simulink model "RoboticFish_Maneuverability_model"  (R2022b)
settings: Solver=ode4  StartTime=0.0  StopTime=50  FixedStep=0.01  RelTol=1e-3  EnableMultiTasking=on
libraries: sharedutil x15, matrix_library x1, dspvision x1, vrlib x1
(part 1 of 3)
settings Model: Creator=Waqas Ali Waqar  LastModifiedBy=Administrator
settings SolverCC: ConcurrentTasks=on  AlgebraicLoopSolver=TrustRegion  AutoInsertRateTranBlk=on  InsertRTBMode=Never (minimum delay)
settings DataIOCC: SaveFormat=StructureWithTime
settings OptimizationCC: BlockReduction=off  OptimizeBlockIOStorage=off  BufferReuse=off  GlobalBufferReuse=off  ExpressionFolding=off  PassReuseOutputArgsThreshold=0  LocalBlockOutputs=off  OptimizeBlockOrder=speed  OptimizeDataStoreBuffers=off  BusAssignmentInplaceUpdate=off
settings DebuggingCC: ParameterTunabilityLossMsg=error  UnconnectedInputMsg=warning  UnconnectedOutputMsg=warning  UnconnectedLineMsg=warning
settings HardwareCC: ProdBitPerPointer=32  ProdBitPerSizeT=32  ProdBitPerPtrDiffT=32  ProdLargestAtomicFloat=None  ProdWordSize=32  ProdLongLongMode=on  ProdHWDeviceType=Generic->32-bit x86 compatible
settings ModelReferenceCC: EnableRefExpFcnMdlSchedulingChecks=on
settings SFSimCC: MATLABDynamicMemAlloc=off  CustomCodeUndefinedFunction=UseInterfaceOnly
settings RTWCC: GenerateReport=on  RTWVerbose=off  LaunchReport=on  RTWCompilerOptimization=on  DLArmComputeVersion=19.05
settings CodeAppCC: ForceParamTrailComments=on  OperatorAnnotations=on
settings GRTTargetCC: TargetLangStandard=C89/C90 (ANSI)

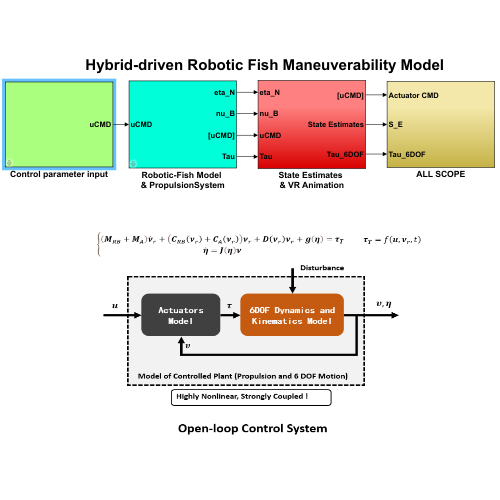
[thumbnail: Simulink's stored preview of the top-level diagram]
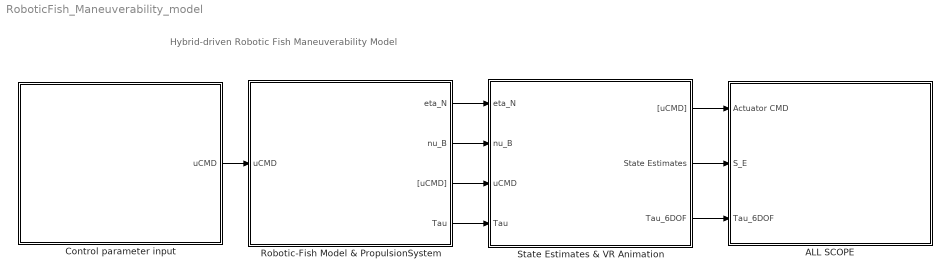
== system RoboticFish_Maneuverability_model ==
  note: Hybrid-driven Robotic Fish Maneuverability Model
  ALL SCOPE : Subsystem
  Control parameter input : Subsystem  mask{PropChoice=on, uHT1=500, uHT2=0, uVT1=1000, FinChoice=off, f_HT3=2, Thetastr_HT3=0, uVT2=60, uVT3=60}
      mask prompts: PropChoice "Choice Propeller Actuators"; uHT1 "uHT1(rpm)"; uHT2 "uHT2(rpm)"; uVT1 "uVT1(rpm)"; FinChoice "Choice Fin Actuators"; f_HT3 "f_HT3(Hz)"; Thetastr_HT3 "Thetastr_HT3(deg)"; uVT2 "uVT2(deg)"; uVT3 "uVT3(deg)"
      mask Callback PropChoice:
      | usePropChoice = get_param(gcbh,'PropChoice');
      | mask_v = get_param(gcbh,'MaskVisibilities');
      | if strcmp('on',usePropChoice)
      |    mask_v{2}='on';
      |    mask_v{3}='on';
      |    mask_v{4}='on';
      | else
      |    mask_v{2}='off';
      |    mask_v{3}='off';
      |    mask_v{4}='off';
      | end
      | set_param(gcbh,'MaskVisibilities',mask_v);
      mask Callback FinChoice:
      | useFinChoice = get_param(gcbh,'FinChoice');
      | mask_v = get_param(gcbh,'MaskVisibilities');
      | if strcmp('on',useFinChoice)
      |    mask_v{6}='on';
      |    mask_v{7}='on';
      |    mask_v{8}='on';
      |    mask_v{9}='on';
      | else
      |    mask_v{6}='off';
      |    mask_v{7}='off';
      |    mask_v{8}='off';
      |    mask_v{9}='off';
      | end
      | set_param(gcbh,'MaskVisibilities',mask_v);
  Robotic-Fish Model & PropulsionSystem : Subsystem  mask{Ig=[0.5025 0 0;0 4.8344 0;0 0 4.9297], m=48, rho=1000, W=470.4, B=470.4, rG_B=[0;0;0], rB_B=[0;0;-0.2], DL=diag([-1.1;2.559;-1.458;0.000811;-0.382;-1.621]), S=0.103, Amp=0.182, ld=0.239, kw=1, a2=1.905, a1=-0.7047, a0=0.01797, b2=2.081, b1=-0.3937, b0=0.09809, c2=20.652, d2=17.102, phisurge=1.0158, phisway=3.792, phiyaw=13.362, cL=0.5, xfin=0.192, yfin=0.225, zfin=0.083, alpha=0, Sfin=0.0121, e1=[1;0;0], r1=[-0.107;-0.222;0], e2=[1;0;0], r2=[-0.107;0.222;0], e3=[0;0;1], r3=[-0.143;0;-0.021], D=0.0762}
      mask prompts: Ig "Inertia Tensor Ig:"; m "Mass m:"; rho "Seawater Density rho:"; W "Weight"; B "Buoyancy"; DL "Linear Damping Matrix"; S "Tail area S (m^2)"; Amp "Tail-beat amplitude Amp (m)"; ld "Distance from the center of hydrodynamic action of the tail to the origin ld (m)"; kw "Adjustment coefficient kw"; cL "fin lift coefficient  cL:"; xfin "fin axial position xfin:"; yfin "fin axial position yfin:"; zfin "fin axial position zfin:"; alpha "fin flutter angle alpha"; Sfin "fin platform area Sfin:"; e1 "e1 (HT1):"; r1 "r1 (HT1):"; e2 "e2 (HT2 ):"; r2 "r2 (HT2):"; e3 "e3 (VT1):"; r3 "r3 (VT1):"; D "Diameter"
      mask init:
      | %%%%%%%%%%%%%%%%%%%%%%%%%%%%%%%%%%%%%%%%%%%%%%%%%%%%%%%
      | %%%%%%%%%%%%%%%%%%%  动力学  %%%%%%%%%%%%%%%%%%%%%%%%
      | %%%%%%%%%%%%%%%%%%%%%%%%%%%%%%%%%%%%%%%%%%%%%%%%%%%%%%%
      | 
      | % 惯性张量与广义质量矩阵
      | Ib = Ig-m*skewsymm(rG_B)*skewsymm(rG_B);
      | MRB = [m*eye(3,3) -m*skewsymm(rG_B); m*skewsymm(rG_B) Ib];
      | 
      | % 附加质量系数
      | X_udot = -7.445;
      | Y_vdot = -63.087;
      | Z_wdot = -63.087;
      | K_pdot = 0;
      | M_qdot = -4.824;
      | N_rdot = -4.824;
      | 
      | 
      | % 附加质量矩阵
      | MA = -diag([X_udot;Y_vdot;Z_wdot;K_pdot;M_qdot;N_rdot]);
      | 
      | % 总的广义质量矩阵（包括附加质量矩阵）
      | M = MRB + MA;
      | inv_M = inv(M);
      | M11 = MA(1:3,1:3);    M12 = MA(1:3,4:6);
      | M21 = MA(4:6,1:3);    M22 = MA(4:6,4:6);
      | 
      | %% 粘性水动力系数
      | X_uu = -3.886;
      | Y_vv = -113;
      | Z_ww = -71.631;
      | K_pp = -0.158;
      | M_qq = -2.127;
      | N_rr = -22.381;
      | 
      | dQ = ([X_uu;Y_vv;Z_ww;K_pp;M_qq;N_rr]);
      | 
      | 
      | %%%%%%%%%%%%%%%%%%%%%%%%%%%%%%%%%%%%%%%%%%%%%%%%%%%%%%%
      | %%%%%%%%%%%%%%%%%%%  PROP HT1 HT2 VT1  %%%%%%%%%%%%%%%%
      | %%%%%%%%%%%%%%%%%%%%%%%%%%%%%%%%%%%%%%%%%%%%%%%%%%%%%%%
      | 
      | K1 = rho*D*D*D;
      | K2 = rho*D*D*D;
      | K3 = rho*D*D*D;
      | HT_prop = [e1 e2;skewsymm(r1)*e1 skewsymm(r2)*e2]*diag([K1;K2]);
      | VT_prop = [e3 ;skewsymm(r3)*e3 ]*K3;
      mask DialogControl DescGroupVar Prompt: Robotic Fish Paramteres
      mask DialogControl Container14 Prompt: Robotic Fish Parameters
      mask DialogControl Container17 Prompt: Caudal Fin Parameters
      mask DialogControl Container18 Prompt: Pectoral Fins Parameters
      mask DialogControl Container19 Prompt: Thrusters Parameters
  State Estimates & VR Animation : Subsystem
  wires:
  Robotic-Fish Model & PropulsionSystem/2(nu_B) -> State Estimates & VR Animation/2(nu_B)
  Robotic-Fish Model & PropulsionSystem/1(eta_N) -> State Estimates & VR Animation/1(eta_N)
  Control parameter input/1(uCMD) -> Robotic-Fish Model & PropulsionSystem/1(uCMD)
  Robotic-Fish Model & PropulsionSystem/3("[uCMD]") -> State Estimates & VR Animation/3(uCMD)
  State Estimates & VR Animation/2(State Estimates) -> ALL SCOPE/2(S_E)
  State Estimates & VR Animation/1("[uCMD]") -> ALL SCOPE/1(Actuator CMD)
  Robotic-Fish Model & PropulsionSystem/4(Tau) -> State Estimates & VR Animation/4(Tau)
  State Estimates & VR Animation/3(Tau_6DOF) -> ALL SCOPE/3(Tau_6DOF)

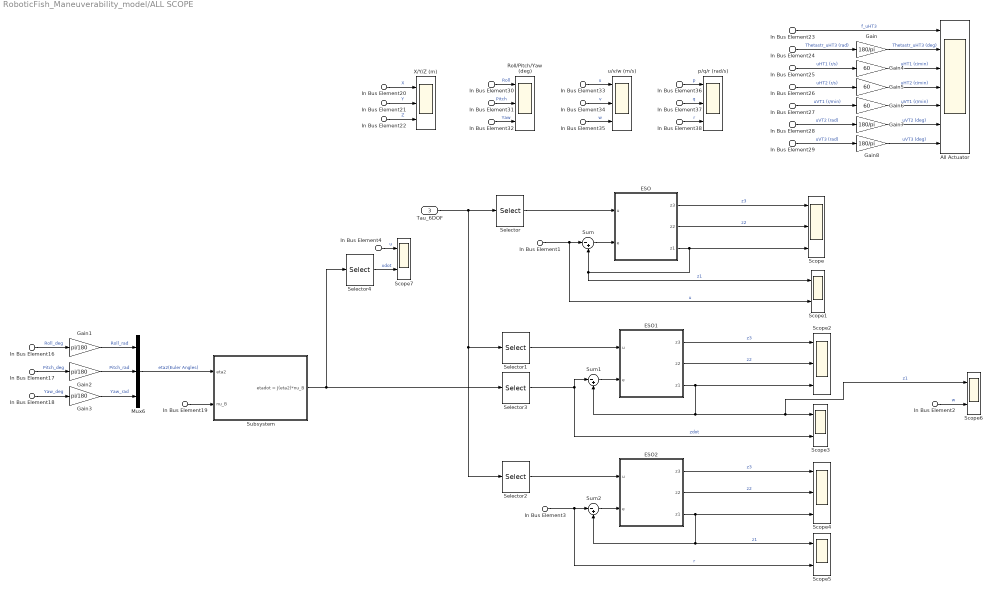
== system RoboticFish_Maneuverability_model/ALL SCOPE ==
  In Bus Element23 : Inport  PortName=Actuator CMD  Element=f_HT3
  In Bus Element24 : Inport  PortName=Actuator CMD  Element=Thetastr_HT3
  In Bus Element25 : Inport  PortName=Actuator CMD  Element=uHT1
  In Bus Element26 : Inport  PortName=Actuator CMD  Element=uHT2
  In Bus Element27 : Inport  PortName=Actuator CMD  Element=uVT1
  In Bus Element29 : Inport  PortName=Actuator CMD  Element=uVT3
  In Bus Element28 : Inport  PortName=Actuator CMD  Element=uVT2
  In Bus Element21 : Inport  Port=2  PortName=S_E  Element=Position.Y
  In Bus Element22 : Inport  Port=2  PortName=S_E  Element=Position.Z
  In Bus Element30 : Inport  Port=2  PortName=S_E  Element=Position.Roll
  In Bus Element16 : Inport  Port=2  PortName=S_E  Element=Position.Roll
  In Bus Element31 : Inport  Port=2  PortName=S_E  Element=Position.Pitch
  In Bus Element17 : Inport  Port=2  PortName=S_E  Element=Position.Pitch
  In Bus Element32 : Inport  Port=2  PortName=S_E  Element=Position.Yaw
  In Bus Element18 : Inport  Port=2  PortName=S_E  Element=Position.Yaw
  In Bus Element20 : Inport  Port=2  PortName=S_E  Element=Position.X
  In Bus Element19 : Inport  Port=2  PortName=S_E  Element=Velocity
  In Bus Element33 : Inport  Port=2  PortName=S_E  Element=Velocity.u
  In Bus Element1 : Inport  Port=2  PortName=S_E  Element=Velocity.u
  In Bus Element4 : Inport  Port=2  PortName=S_E  Element=Velocity.u
  In Bus Element34 : Inport  Port=2  PortName=S_E  Element=Velocity.v
  In Bus Element35 : Inport  Port=2  PortName=S_E  Element=Velocity.w
  In Bus Element2 : Inport  Port=2  PortName=S_E  Element=Velocity.w
  In Bus Element36 : Inport  Port=2  PortName=S_E  Element=Velocity.p
  In Bus Element37 : Inport  Port=2  PortName=S_E  Element=Velocity.q
  In Bus Element38 : Inport  Port=2  PortName=S_E  Element=Velocity.r
  In Bus Element3 : Inport  Port=2  PortName=S_E  Element=Velocity.r
  Tau_6DOF : Inport  Port=3
  All Actuator : Scope  NumInputPorts=7
  ESO : Subsystem  mask(ESO){h=0.01, beta_01=100, beta_02=500, beta_03=1500, b0=1}
      mask help: 这一部分（扩张状态观测器）的作用是得到系统状态变量的估计值及扩张状态的实时作用量。
      mask Display: disp('ESO');
  ESO1 : Subsystem  mask(ESO){h=0.01, beta_01=100, beta_02=300, beta_03=1000, b0=1}
      mask help: 这一部分（扩张状态观测器）的作用是得到系统状态变量的估计值及扩张状态的实时作用量。
      mask Display: disp('ESO');
  ESO2 : Subsystem  mask(ESO){h=0.01, beta_01=100, beta_02=1800, beta_03=3000, b0=1}
      mask help: 这一部分（扩张状态观测器）的作用是得到系统状态变量的估计值及扩张状态的实时作用量。
      mask Display: disp('ESO');
  Gain : Gain  Gain=180/pi
  Gain1 : Gain  Gain=pi/180
  Gain2 : Gain  Gain=pi/180
  Gain3 : Gain  Gain=pi/180
  Gain4 : Gain  Gain=60
  Gain5 : Gain  Gain=60
  Gain6 : Gain  Gain=60
  Gain7 : Gain  Gain=180/pi
  Gain8 : Gain  Gain=180/pi
  Mux6 : Mux  Inputs=3
  Roll/Pitch/Yaw (deg) : Scope  NumInputPorts=3
  Scope : Scope  NumInputPorts=3
  Scope{1,3,5..7} (5 alike) : Scope  NumInputPorts=2
  Scope2 : Scope  NumInputPorts=3
  Scope4 : Scope  NumInputPorts=3
  Selector : Selector  InputPortWidth=6  IndexOptions=Index vector (dialog)  Indices=[1]  OutputSizes=1
  Selector1 : Selector  InputPortWidth=6  IndexOptions=Index vector (dialog)  Indices=[3]  OutputSizes=1
  Selector2 : Selector  InputPortWidth=6  IndexOptions=Index vector (dialog)  Indices=[6]  OutputSizes=1
  Selector3 : Selector  InputPortWidth=6  IndexOptions=Index vector (dialog)  Indices=[3]  OutputSizes=1
  Selector4 : Selector  InputPortWidth=6  IndexOptions=Index vector (dialog)  Indices=[1]  OutputSizes=1
  Subsystem : Subsystem
  Sum : Sum  Inputs=|-+
  Sum1 : Sum  Inputs=|-+
  Sum2 : Sum  Inputs=|-+
  X/Y/Z (m) : Scope  NumInputPorts=3
  p/q/r (rad/s) : Scope  NumInputPorts=3
  u/v/w (m/s) : Scope  NumInputPorts=3
  wires:
  In Bus Element29/1 -> Gain8/1  "uVT3 (rad)"
  In Bus Element26/1 -> Gain5/1  "uHT2 (r/s)"
  In Bus Element24/1 -> Gain/1  "Thetastr_uHT3 (rad)"
  In Bus Element23/1 -> All Actuator/1  "f_uHT3"
  In Bus Element25/1 -> Gain4/1  "uHT1 (r/s)"
  In Bus Element28/1 -> Gain7/1  "uVT2 (rad)"
  In Bus Element27/1 -> Gain6/1  "uVT1 (r/min)"
  In Bus Element20/1 -> X/Y/Z (m)/1  "X"
  In Bus Element21/1 -> X/Y/Z (m)/2  "Y"
  In Bus Element22/1 -> X/Y/Z (m)/3  "Z"
  In Bus Element30/1 -> Roll/Pitch/Yaw (deg)/1  "Roll"
  In Bus Element31/1 -> Roll/Pitch/Yaw (deg)/2  "Pitch"
  In Bus Element32/1 -> Roll/Pitch/Yaw (deg)/3  "Yaw"
  In Bus Element33/1 -> u/v/w (m/s)/1  "u"
  In Bus Element34/1 -> u/v/w (m/s)/2  "v"
  In Bus Element35/1 -> u/v/w (m/s)/3  "w"
  In Bus Element36/1 -> p/q/r (rad/s)/1  "p"
  In Bus Element37/1 -> p/q/r (rad/s)/2  "q"
  In Bus Element38/1 -> p/q/r (rad/s)/3  "r"
  Gain/1 -> All Actuator/2  "Thetastr_uHT3 (deg)"
  Gain4/1 -> All Actuator/3  "uHT1 (r/min)"
  Gain5/1 -> All Actuator/4  "uHT2 (r/min)"
  Gain6/1 -> All Actuator/5  "uVT1 (r/min)"
  Gain7/1 -> All Actuator/6  "uVT2 (deg)"
  Gain8/1 -> All Actuator/7  "uVT3 (deg)"
  Selector/1 -> ESO/1(u)
  In Bus Element1/1 -> Scope1/2, Sum/1  "u"
  ESO/3(z1) -> Scope1/1, Sum/2, Scope/3  "z1"
  ESO/2(z2) -> Scope/2  "z2"
  ESO/1(z3) -> Scope/1  "z3"
  Sum/1 -> ESO/2(e)
  Sum1/1 -> ESO1/2(e)
  ESO1/1(z3) -> Scope2/1  "z3"
  ESO1/2(z2) -> Scope2/2  "z2"
  ESO1/3(z1) -> Scope2/3, Sum1/2, Scope6/1, Scope3/1  "z1"
  Selector3/1 -> Sum1/1, Scope3/2  "zdot"
  Selector1/1 -> ESO1/1(u)
  Selector2/1 -> ESO2/1(u)
  In Bus Element3/1 -> Scope5/2, Sum2/1  "r"
  ESO2/3(z1) -> Scope5/1, Sum2/2, Scope4/3  "z1"
  ESO2/2(z2) -> Scope4/2  "z2"
  ESO2/1(z3) -> Scope4/1  "z3"
  Sum2/1 -> ESO2/2(e)
  Tau_6DOF/1 -> Selector2/1, Selector1/1, Selector/1
  In Bus Element16/1 -> Gain1/1  "Roll_deg"
  In Bus Element18/1 -> Gain3/1  "Yaw_deg"
  Subsystem/1(etadot = J(eta2)*nu_B) -> Selector4/1, Selector3/1
  Gain3/1 -> Mux6/3  "Yaw_rad"
  Gain1/1 -> Mux6/1  "Roll_rad"
  In Bus Element19/1 -> Subsystem/2(nu_B)
  Mux6/1 -> Subsystem/1(eta2)  "eta2(Euler Angles)"
  In Bus Element17/1 -> Gain2/1  "Pitch_deg"
  Gain2/1 -> Mux6/2  "Pitch_rad"
  In Bus Element2/1 -> Scope6/2  "w"
  Selector4/1 -> Scope7/2  "xdot"
  In Bus Element4/1 -> Scope7/1  "u"

== system RoboticFish_Maneuverability_model/Control parameter input ==
  Constant7 : Constant  Value=FinChoice
  Constant8 : Constant  Value=PropChoice
  Subsystem : Subsystem
  uCMD : Outport  VectorParamsAs1DForOutWhenUnconnected=off
  wires:
  Constant8/1 -> Subsystem/1(In1)
  Constant7/1 -> Subsystem/2(In2)
  Subsystem/1(f_HT3 Thetastr_HT3 uHT1 uHT2 uVT1 uVT2 uVT3) -> uCMD/1

== system RoboticFish_Maneuverability_model/Robotic-Fish Model & PropulsionSystem ==
  uCMD : Inport
  Memory : Memory
  Propulsion System : Subsystem
  RF Dynamics and Kinematics (Attitude rappresentation: Quaternions) : Subsystem
      mask Display: image('坐标系.jpg'); % 使用工具条上的 "编辑图像" 进行更改。
  Subsystem : Subsystem
  eta_N : Outport  VectorParamsAs1DForOutWhenUnconnected=off
  nu_B : Outport  Port=2  VectorParamsAs1DForOutWhenUnconnected=off
  "[uCMD]" : Outport  Port=3
  Tau : Outport  Port=4
  wires:
  RF Dynamics and Kinematics (Attitude rappresentation: Quaternions)/2(eta_N) -> eta_N/1  "[x   y   z  q0  q1  q2  q3]"
  Memory/1 -> Propulsion System/1(nu_B)
  RF Dynamics and Kinematics (Attitude rappresentation: Quaternions)/1(nu_B) -> Memory/1, nu_B/1  "[u    v    w    p    q    r]"
  uCMD/1 -> "[uCMD]"/1, Propulsion System/2(uCMD)
  Propulsion System/1(Tau_B) -> Subsystem/1("[Tau_X Tau_Y  Tau_Z  Tau_Roll  Tau_Pitch Tau_Yaw]"), Tau/1, RF Dynamics and Kinematics (Attitude rappresentation: Quaternions)/1(tau_B)  "[Tau_X Tau_Y  Tau_Z  Tau_Roll  Tau_Pitch Tau_Yaw]"

== system RoboticFish_Maneuverability_model/State Estimates & VR Animation ==
  eta_N : Inport
  nu_B : Inport  Port=2
  uCMD : Inport  Port=3
  Tau : Inport  Port=4
  Gain : Gain  Gain=180/pi
  Mux : Mux  Inputs=2
  Quaternions to Euler Angles : Subsystem
  VR sink : Subsystem
  eta1_E=[x,y,z] : Selector  InputPortWidth=7  IndexOptions=Index vector (dialog)  Indices=[1 2 3]  OutputSizes=1
  eta2_E=[q0,q1,q2,q3] : Selector  InputPortWidth=7  IndexOptions=Index vector (dialog)  Indices=[4 5 6 7]  OutputSizes=1
  signal transformation1 : Subsystem
  "[uCMD]" : Outport  VectorParamsAs1DForOutWhenUnconnected=off
  State Estimates : Outport  Port=2  VectorParamsAs1DForOutWhenUnconnected=off
  Tau_6DOF : Outport  Port=3
  wires:
  Gain/1 -> Mux/2
  signal transformation1/1(State Estimate) -> State Estimates/1
  eta1_E=[x,y,z]/1 -> Mux/1
  Quaternions to Euler Angles/1(Euler Angles) -> Gain/1
  Mux/1 -> signal transformation1/1(Position)
  eta2_E=[q0,q1,q2,q3]/1 -> Quaternions to Euler Angles/1(Quaternions)
  nu_B/1 -> signal transformation1/2(nu_B)
  eta_N/1 -> VR sink/2(eta_N), eta1_E=[x,y,z]/1, eta2_E=[q0,q1,q2,q3]/1  "[x   y   z  q0  q1  q2  q3]"
  uCMD/1 -> "[uCMD]"/1, VR sink/1(uCMD)
  Tau/1 -> Tau_6DOF/1

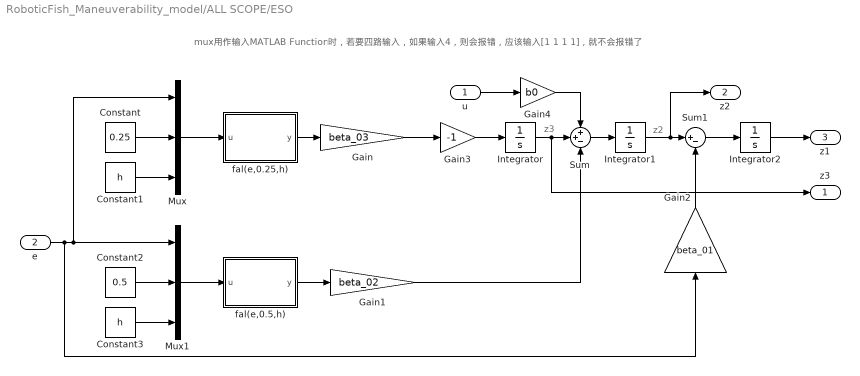
== system RoboticFish_Maneuverability_model/ALL SCOPE/ESO ==
  note: z2
  note: z3
  note: mux用作输入MATLAB Function时，若要四路输入，如果输入4，则会报错，应该输入[1 1 1 1]，就不会报错了
  u : Inport
  e : Inport  Port=2
  Constant : Constant  Value=0.25
  Constant1 : Constant  Value=h
  Constant2 : Constant  Value=0.5
  Constant3 : Constant  Value=h
  Gain : Gain  Gain=beta_03
  Gain1 : Gain  Gain=beta_02
  Gain2 : Gain  Gain=beta_01
  Gain3 : Gain  Gain=-1
  Gain4 : Gain  Gain=b0
  Integrator : Integrator
  Integrator1 : Integrator
  Integrator2 : Integrator
  Mux : Mux  Inputs=[1 1 1]
  Mux1 : Mux  Inputs=[1 1 1]
  Sum : Sum  Inputs=++-
  Sum1 : Sum  Inputs=|+-
  fal(e,0.25,h) : MATLAB Function  TreatAsAtomicUnit=on
  fal(e,0.5,h) : MATLAB Function  TreatAsAtomicUnit=on
  z3 : Outport  VectorParamsAs1DForOutWhenUnconnected=off
  z2 : Outport  Port=2  VectorParamsAs1DForOutWhenUnconnected=off
  z1 : Outport  Port=3  VectorParamsAs1DForOutWhenUnconnected=off
  wires:
  Mux1/1 -> fal(e,0.5,h)/1(u)
  Mux/1 -> fal(e,0.25,h)/1(u)
  e/1 -> Gain2/1, Mux/1, Mux1/1
  Constant1/1 -> Mux/3
  Sum/1 -> Integrator1/1
  Gain2/1 -> Sum1/2
  Constant2/1 -> Mux1/2
  Gain4/1 -> Sum/1
  Integrator/1 -> z3/1, Sum/2
  fal(e,0.25,h)/1(y) -> Gain/1
  u/1 -> Gain4/1
  Gain1/1 -> Sum/3
  Constant3/1 -> Mux1/3
  Constant/1 -> Mux/2
  Integrator1/1 -> z2/1, Sum1/1
  Gain/1 -> Gain3/1
  Gain3/1 -> Integrator/1
  Sum1/1 -> Integrator2/1
  fal(e,0.5,h)/1(y) -> Gain1/1
  Integrator2/1 -> z1/1

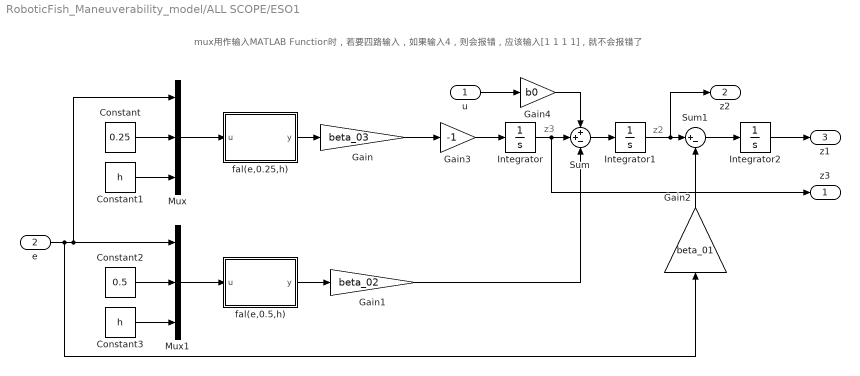
== system RoboticFish_Maneuverability_model/ALL SCOPE/ESO1 ==
  note: mux用作输入MATLAB Function时，若要四路输入，如果输入4，则会报错，应该输入[1 1 1 1]，就不会报错了
  note: z3
  note: z2
  u : Inport
  e : Inport  Port=2
  Constant : Constant  Value=0.25
  Constant1 : Constant  Value=h
  Constant2 : Constant  Value=0.5
  Constant3 : Constant  Value=h
  Gain : Gain  Gain=beta_03
  Gain1 : Gain  Gain=beta_02
  Gain2 : Gain  Gain=beta_01
  Gain3 : Gain  Gain=-1
  Gain4 : Gain  Gain=b0
  Integrator : Integrator
  Integrator1 : Integrator
  Integrator2 : Integrator
  Mux : Mux  Inputs=[1 1 1]
  Mux1 : Mux  Inputs=[1 1 1]
  Sum : Sum  Inputs=++-
  Sum1 : Sum  Inputs=|+-
  fal(e,0.25,h) : MATLAB Function  TreatAsAtomicUnit=on
  fal(e,0.5,h) : MATLAB Function  TreatAsAtomicUnit=on
  z3 : Outport  VectorParamsAs1DForOutWhenUnconnected=off
  z2 : Outport  Port=2  VectorParamsAs1DForOutWhenUnconnected=off
  z1 : Outport  Port=3  VectorParamsAs1DForOutWhenUnconnected=off
  wires:
  Integrator2/1 -> z1/1
  fal(e,0.5,h)/1(y) -> Gain1/1
  Sum1/1 -> Integrator2/1
  Gain3/1 -> Integrator/1
  Gain/1 -> Gain3/1
  Integrator1/1 -> Sum1/1, z2/1
  Constant/1 -> Mux/2
  Constant3/1 -> Mux1/3
  Gain1/1 -> Sum/3
  u/1 -> Gain4/1
  fal(e,0.25,h)/1(y) -> Gain/1
  Integrator/1 -> Sum/2, z3/1
  Gain4/1 -> Sum/1
  Constant2/1 -> Mux1/2
  Gain2/1 -> Sum1/2
  Sum/1 -> Integrator1/1
  Constant1/1 -> Mux/3
  e/1 -> Mux1/1, Mux/1, Gain2/1
  Mux/1 -> fal(e,0.25,h)/1(u)
  Mux1/1 -> fal(e,0.5,h)/1(u)

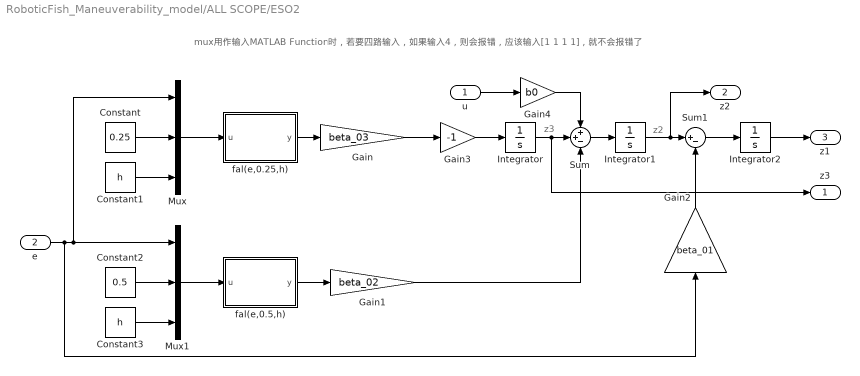
== system RoboticFish_Maneuverability_model/ALL SCOPE/ESO2 ==
  note: z2
  note: z3
  note: mux用作输入MATLAB Function时，若要四路输入，如果输入4，则会报错，应该输入[1 1 1 1]，就不会报错了
  u : Inport
  e : Inport  Port=2
  Constant : Constant  Value=0.25
  Constant1 : Constant  Value=h
  Constant2 : Constant  Value=0.5
  Constant3 : Constant  Value=h
  Gain : Gain  Gain=beta_03
  Gain1 : Gain  Gain=beta_02
  Gain2 : Gain  Gain=beta_01
  Gain3 : Gain  Gain=-1
  Gain4 : Gain  Gain=b0
  Integrator : Integrator
  Integrator1 : Integrator
  Integrator2 : Integrator
  Mux : Mux  Inputs=[1 1 1]
  Mux1 : Mux  Inputs=[1 1 1]
  Sum : Sum  Inputs=++-
  Sum1 : Sum  Inputs=|+-
  fal(e,0.25,h) : MATLAB Function  TreatAsAtomicUnit=on
  fal(e,0.5,h) : MATLAB Function  TreatAsAtomicUnit=on
  z3 : Outport  VectorParamsAs1DForOutWhenUnconnected=off
  z2 : Outport  Port=2  VectorParamsAs1DForOutWhenUnconnected=off
  z1 : Outport  Port=3  VectorParamsAs1DForOutWhenUnconnected=off
  wires:
  Mux1/1 -> fal(e,0.5,h)/1(u)
  Mux/1 -> fal(e,0.25,h)/1(u)
  e/1 -> Gain2/1, Mux/1, Mux1/1
  Constant1/1 -> Mux/3
  Sum/1 -> Integrator1/1
  Gain2/1 -> Sum1/2
  Constant2/1 -> Mux1/2
  Gain4/1 -> Sum/1
  Integrator/1 -> z3/1, Sum/2
  fal(e,0.25,h)/1(y) -> Gain/1
  u/1 -> Gain4/1
  Gain1/1 -> Sum/3
  Constant3/1 -> Mux1/3
  Constant/1 -> Mux/2
  Integrator1/1 -> z2/1, Sum1/1
  Gain/1 -> Gain3/1
  Gain3/1 -> Integrator/1
  Sum1/1 -> Integrator2/1
  fal(e,0.5,h)/1(y) -> Gain1/1
  Integrator2/1 -> z1/1

== system RoboticFish_Maneuverability_model/ALL SCOPE/Subsystem ==
  note: u v w
  note: p q r
  eta2 : Inport
  nu_B : Inport  Port=2
  Bus Creator : BusCreator  Inputs=6
  J1 : Subsystem
  J2 : Subsystem
  Product2 : Product  Inputs=**  Multiplication=Matrix(*)  SaturateOnIntegerOverflow=on  OutDataTypeStr=Inherit: Same as first input
  Product3 : Product  Inputs=**  Multiplication=Matrix(*)  SaturateOnIntegerOverflow=on  OutDataTypeStr=Inherit: Same as first input
  Selector1 : Selector  InputPortWidth=3  IndexOptions=Index vector (dialog)  Indices=[2]  OutputSizes=1
  Selector2 : Selector  InputPortWidth=6  IndexOptions=Index vector (dialog)  Indices=[1 2 3]  OutputSizes=1
  Selector3 : Selector  InputPortWidth=3  IndexOptions=Index vector (dialog)  Indices=[1]  OutputSizes=1
  Selector4 : Selector  InputPortWidth=6  IndexOptions=Index vector (dialog)  Indices=[4 5 6]  OutputSizes=1
  Selector5 : Selector  InputPortWidth=3  IndexOptions=Index vector (dialog)  Indices=[3]  OutputSizes=1
  Selector6 : Selector  InputPortWidth=3  IndexOptions=Index vector (dialog)  Indices=[1]  OutputSizes=1
  Selector7 : Selector  InputPortWidth=3  IndexOptions=Index vector (dialog)  Indices=[2]  OutputSizes=1
  Selector8 : Selector  InputPortWidth=3  IndexOptions=Index vector (dialog)  Indices=[3]  OutputSizes=1
  etadot = J(eta2)*nu_B : Outport
  wires:
  eta2/1 -> J1/1(eta2), J2/1(eta2)
  J1/1(J1) -> Product2/1
  J2/1(J2) -> Product3/1
  nu_B/1 -> Selector4/1, Selector2/1
  Selector4/1 -> Product3/2
  Selector2/1 -> Product2/2
  Product2/1 -> Selector5/1, Selector1/1, Selector3/1  "eta1dot"
  Product3/1 -> Selector8/1, Selector7/1, Selector6/1  "eta2dot(Euler Angles)"
  Bus Creator/1 -> etadot = J(eta2)*nu_B/1
  Selector3/1 -> Bus Creator/1  "xdot"
  Selector1/1 -> Bus Creator/2  "ydot"
  Selector5/1 -> Bus Creator/3  "zdot"
  Selector6/1 -> Bus Creator/4  "rolldot"
  Selector7/1 -> Bus Creator/5  "pitchdot"
  Selector8/1 -> Bus Creator/6  "yawdot"

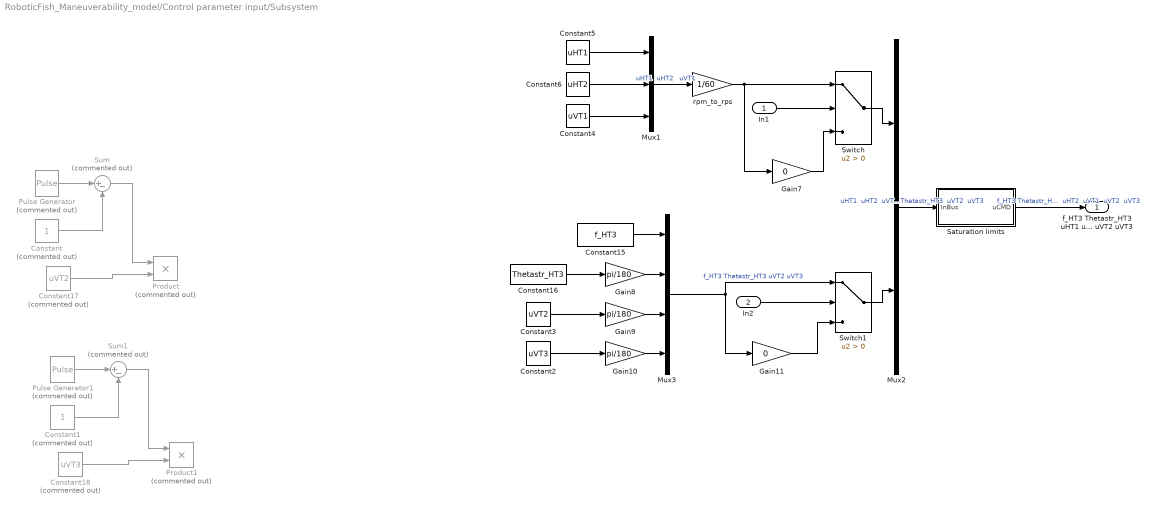
== system RoboticFish_Maneuverability_model/Control parameter input/Subsystem ==
  In1 : Inport
  In2 : Inport  Port=2
  Constant : Constant  Commented=on
  Constant1 : Constant  Commented=on
  Constant15 : Constant  Value=f_HT3
  Constant16 : Constant  Value=Thetastr_HT3
  Constant17 : Constant  Commented=on  Value=uVT2
  Constant18 : Constant  Commented=on  Value=uVT3
  Constant2 : Constant  Value=uVT3
  Constant3 : Constant  Value=uVT2
  Constant4 : Constant  Value=uVT1
  Constant5 : Constant  Value=uHT1
  Constant6 : Constant  Value=uHT2
  Gain10 : Gain  Gain=pi/180
  Gain11 : Gain  Gain=0
  Gain7 : Gain  Gain=0
  Gain8 : Gain  Gain=pi/180
  Gain9 : Gain  Gain=pi/180
  Mux1 : Mux  Inputs=3
  Mux2 : Mux  Inputs=2
  Mux3 : Mux
  Product : Product  Commented=on
  Product1 : Product  Commented=on
  Pulse Generator : DiscretePulseGenerator  Commented=on  PulseType=Time based  Amplitude=2  Period=100  PulseWidth=50
  Pulse Generator1 : DiscretePulseGenerator  Commented=on  PulseType=Time based  Amplitude=2  Period=100  PulseWidth=50
  Saturation limits : Subsystem
  Sum : Sum  Commented=on  Inputs=|+-
  Sum1 : Sum  Commented=on  Inputs=|+-
  Switch : Switch  Criteria=u2 > Threshold  SaturateOnIntegerOverflow=off  InputSameDT=off
  Switch1 : Switch  Criteria=u2 > Threshold  SaturateOnIntegerOverflow=off  InputSameDT=off
  rpm_to_rps : Gain  Gain=1/60
  f_HT3 Thetastr_HT3 uHT1 uHT2 uVT1 uVT2 uVT3 : Outport
  wires:
  Constant5/1 -> Mux1/1
  Constant6/1 -> Mux1/2
  rpm_to_rps/1 -> Gain7/1, Switch/1
  Gain7/1 -> Switch/3
  Mux1/1 -> rpm_to_rps/1  "uHT1  uHT2   uVT1"
  Mux3/1 -> Gain11/1, Switch1/1  "f_HT3 Thetastr_HT3 uVT2 uVT3"
  Gain11/1 -> Switch1/3
  Gain8/1 -> Mux3/2
  Gain10/1 -> Mux3/4
  Saturation limits/1(uCMD) -> f_HT3 Thetastr_HT3 uHT1 uHT2 uVT1 uVT2 uVT3/1  "f_HT3 Thetastr_HT3  uHT1  uHT2  uVT1  uVT2  uVT3"
  Switch1/1 -> Mux2/2
  Constant4/1 -> Mux1/3
  Gain9/1 -> Mux3/3
  Mux2/1 -> Saturation limits/1(InBus)  "uHT1  uHT2  uVT1 f_HT3 Thetastr_HT3  uVT2  uVT3"
  In2/1 -> Switch1/2
  Switch/1 -> Mux2/1
  In1/1 -> Switch/2
  Pulse Generator/1 -> Sum/1
  Constant/1 -> Sum/2
  Sum/1 -> Product/1
  Constant17/1 -> Product/2
  Constant1/1 -> Sum1/2
  Sum1/1 -> Product1/1
  Pulse Generator1/1 -> Sum1/1
  Constant18/1 -> Product1/2
  Constant3/1 -> Gain9/1
  Constant2/1 -> Gain10/1
  Constant15/1 -> Mux3/1
  Constant16/1 -> Gain8/1

== system RoboticFish_Maneuverability_model/Robotic-Fish Model & PropulsionSystem/Propulsion System ==
  note: square
  nu_B : Inport
  In Bus Element1 : Inport  Port=2  PortName=uCMD  Element=f_HT3
  In Bus Element4 : Inport  Port=2  PortName=uCMD  Element=uHT2
  In Bus Element5 : Inport  Port=2  PortName=uCMD  Element=uVT1
  In Bus Element6 : Inport  Port=2  PortName=uCMD  Element=uVT2
  In Bus Element7 : Inport  Port=2  PortName=uCMD  Element=uVT3
  In Bus Element8 : Inport  Port=2  PortName=uCMD  Element=Thetastr_HT3
  In Bus Element2 : Inport  Port=2  PortName=uCMD  Element=uHT1
  Bus Creator : BusCreator  Inputs=2
  Bus Creator1 : BusCreator  Inputs=2
  Horizontal Force and Moment (Tau_H) : Subsystem
  Sum : Sum  Inputs=|++
  Vertical Force and Moment (Tau_V) : Subsystem
  Tau_B : Outport  VectorParamsAs1DForOutWhenUnconnected=off
  wires:
  nu_B/1 -> Vertical Force and Moment (Tau_V)/1(nu_B), Horizontal Force and Moment (Tau_H)/4(nu_B)
  Horizontal Force and Moment (Tau_H)/1(Horizontal _Tau) -> Sum/1
  Vertical Force and Moment (Tau_V)/1(Vertical_Tau) -> Sum/2
  In Bus Element6/1 -> Bus Creator/1
  In Bus Element7/1 -> Bus Creator/2
  Bus Creator/1 -> Vertical Force and Moment (Tau_V)/3("[uVT2 uVT3]")
  In Bus Element5/1 -> Vertical Force and Moment (Tau_V)/2(uVT1)
  In Bus Element4/1 -> Horizontal Force and Moment (Tau_H)/3(uHT2)
  In Bus Element2/1 -> Horizontal Force and Moment (Tau_H)/2(uHT1)
  In Bus Element1/1 -> Bus Creator1/1
  In Bus Element8/1 -> Bus Creator1/2
  Bus Creator1/1 -> Horizontal Force and Moment (Tau_H)/1(uHT3)
  Sum/1 -> Tau_B/1  "[Tau_X, Tau_Y, Tau_Z, Tau_Roll, Tau_Pitch, Tau_Yaw]"

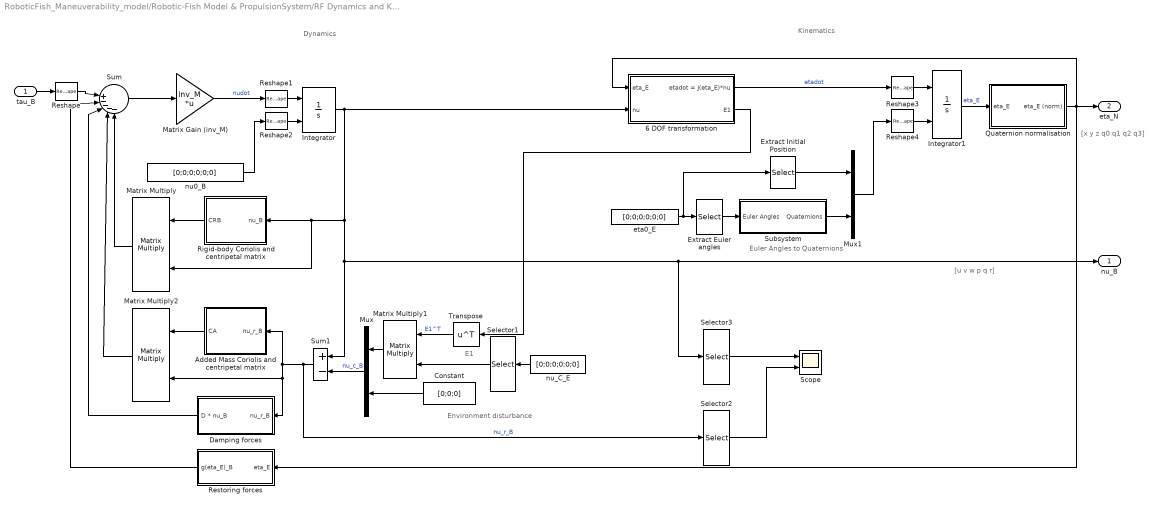
== system RoboticFish_Maneuverability_model/Robotic-Fish Model & PropulsionSystem/RF Dynamics and Kinematics (Attitude rappresentation: Quaternions) ==
  note: Kinematics
  note: E1
  note: Euler Angles to Quaternions
  note: [x y z q0 q1 q2 q3]
  note: [u v w p q r]
  note: Environment disturbance
  note: Dynamics
  tau_B : Inport
  6 DOF transformation : Subsystem
  Added Mass Coriolis and centripetal matrix : Subsystem
  Constant : Constant  Value=[0;0;0]
  Damping forces : Subsystem
  Extract Euler angles : Selector  InputPortWidth=6  IndexOptions=Index vector (dialog)  Indices=[4 5 6]  OutputSizes=1
  Extract Initial Position : Selector  InputPortWidth=6  IndexOptions=Index vector (dialog)  Indices=[1 2 3]  OutputSizes=1
  Integrator : Integrator  InitialConditionSource=external
  Integrator1 : Integrator  InitialConditionSource=external
  Matrix Gain (inv_M) : Gain  Gain=inv_M  Multiplication=Matrix(K*u)  SaturateOnIntegerOverflow=on  OutDataTypeStr=Inherit: Same as input  ParamDataTypeStr=Inherit: Same as input
  Matrix Multiply : Product  Multiplication=Matrix(*)
  Matrix Multiply1 : Product  Multiplication=Matrix(*)
  Matrix Multiply2 : Product  Multiplication=Matrix(*)
  Mux : Mux  Inputs=2
  Mux1 : Mux  Inputs=2
  Quaternion normalisation : Subsystem
  Reshape{,1..4} (5 alike) : Reshape  OutputDimensionality=Column vector (2-D)
  Restoring forces : Subsystem
  Rigid-body Coriolis and centripetal matrix : Subsystem
  Scope : Scope  NumInputPorts=2
  Selector1 : Selector  InputPortWidth=6  IndexOptions=Index vector (dialog)  Indices=[1 2 3]  OutputSizes=1
  Selector2 : Selector  InputPortWidth=6  IndexOptions=Index vector (dialog)  Indices=[1]  OutputSizes=1
  Selector3 : Selector  InputPortWidth=6  IndexOptions=Index vector (dialog)  Indices=[1]  OutputSizes=1
  Subsystem : Subsystem
  Sum : Sum  Inputs=|||+----  SaturateOnIntegerOverflow=on
  Sum1 : Sum  Inputs=+-
  Transpose : Math  Operator=transpose  SignedPower=on
  eta0_E : Constant  Value=[0;0;0;0;0;0]
  nu0_B : Constant  Value=[0;0;0;0;0;0]
  nu_C_E : Constant  Value=[0;0;0;0;0;0]
  nu_B : Outport  VectorParamsAs1DForOutWhenUnconnected=off
  eta_N : Outport  Port=2  VectorParamsAs1DForOutWhenUnconnected=off
  wires:
  Subsystem/1(Quaternions) -> Mux1/2
  Restoring forces/1(g(eta_E)_B) -> Sum/2
  eta0_E/1 -> Extract Initial Position/1, Extract Euler angles/1
  Extract Initial Position/1 -> Mux1/1
  Selector1/1 -> Matrix Multiply1/2
  Matrix Gain (inv_M)/1 -> Reshape1/1  "nudot"
  Reshape4/1 -> Integrator1/2
  tau_B/1 -> Reshape/1
  Constant/1 -> Mux/2
  Quaternion normalisation/1(eta_E (norm)) -> 6 DOF transformation/1(eta_E), eta_N/1, Restoring forces/1(eta_E)
  Mux1/1 -> Reshape4/1
  nu_C_E/1 -> Selector1/1
  Extract Euler angles/1 -> Subsystem/1("Euler Angles ")
  Reshape/1 -> Sum/1
  Reshape1/1 -> Integrator/1
  Damping forces/1(D * nu_B) -> Sum/3
  Integrator1/1 -> Quaternion normalisation/1(eta_E)  "eta_E"
  6 DOF transformation/2(E1) -> Transpose/1
  Sum/1 -> Matrix Gain (inv_M)/1
  Rigid-body Coriolis and centripetal matrix/1(CRB) -> Matrix Multiply/1
  Mux/1 -> Sum1/2  "nu_c_B"
  6 DOF transformation/1(etadot = J(eta_E)*nu) -> Reshape3/1  "etadot"
  Integrator/1 -> Matrix Multiply/2, Rigid-body Coriolis and centripetal matrix/1(nu_B), Sum1/1, Selector3/1, nu_B/1, 6 DOF transformation/2(nu)
  Matrix Multiply/1 -> Sum/5
  Transpose/1 -> Matrix Multiply1/1  "E1^T"
  Matrix Multiply1/1 -> Mux/1
  Sum1/1 -> Selector2/1, Damping forces/1(nu_r_B), Matrix Multiply2/2, Added Mass Coriolis and centripetal matrix/1(nu_r_B)  "nu_r_B"
  nu0_B/1 -> Reshape2/1
  Added Mass Coriolis and centripetal matrix/1(CA) -> Matrix Multiply2/1
  Reshape2/1 -> Integrator/2
  Matrix Multiply2/1 -> Sum/4
  Reshape3/1 -> Integrator1/1
  Selector2/1 -> Scope/2
  Selector3/1 -> Scope/1

== system RoboticFish_Maneuverability_model/Robotic-Fish Model & PropulsionSystem/Subsystem ==
  "[Tau_X Tau_Y  Tau_Z  Tau_Roll  Tau_Pitch Tau_Yaw]" : Inport
  6dof Tau : Scope  NumInputPorts=6
  Selector1 : Selector  InputPortWidth=6  IndexOptions=Index vector (dialog)  Indices=[3]  OutputSizes=1
  Selector2 : Selector  InputPortWidth=6  IndexOptions=Index vector (dialog)  Indices=[4]  OutputSizes=1
  Selector3 : Selector  InputPortWidth=6  IndexOptions=Index vector (dialog)  Indices=[1]  OutputSizes=1
  Selector4 : Selector  InputPortWidth=6  IndexOptions=Index vector (dialog)  Indices=[5]  OutputSizes=1
  Selector5 : Selector  InputPortWidth=6  IndexOptions=Index vector (dialog)  Indices=[2]  OutputSizes=1
  Selector8 : Selector  InputPortWidth=6  IndexOptions=Index vector (dialog)  Indices=[6]  OutputSizes=1
  To Workspace1 : ToWorkspace  VariableName=Tau_Surge  SampleTime=-1
  To Workspace2 : ToWorkspace  VariableName=Tau_Sway  SampleTime=-1
  To Workspace3 : ToWorkspace  VariableName=Tau_Heave  SampleTime=-1
  To Workspace4 : ToWorkspace  VariableName=Tau_Roll  SampleTime=-1
  To Workspace5 : ToWorkspace  VariableName=Tau_Pitch  SampleTime=-1
  To Workspace6 : ToWorkspace  VariableName=Tau_Yaw  SampleTime=-1
  wires:
  "[Tau_X Tau_Y  Tau_Z  Tau_Roll  Tau_Pitch Tau_Yaw]"/1 -> Selector4/1, Selector2/1, Selector1/1, Selector3/1, Selector5/1, Selector8/1
  Selector3/1 -> To Workspace1/1, 6dof Tau/1  "Tau_X"
  Selector4/1 -> To Workspace5/1, 6dof Tau/5  "Tau_Pitch"
  Selector8/1 -> To Workspace6/1, 6dof Tau/6  "Tau_Yaw"
  Selector5/1 -> To Workspace2/1, 6dof Tau/2  "Tau_Y"
  Selector1/1 -> To Workspace3/1, 6dof Tau/3  "Tau_Z"
  Selector2/1 -> 6dof Tau/4, To Workspace4/1  "Tau_Roll"

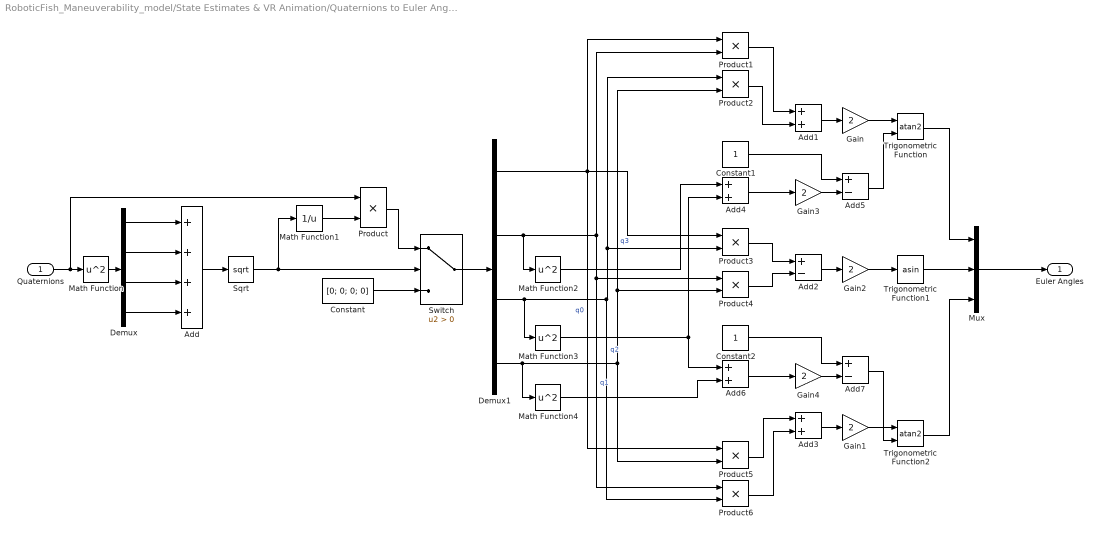
== system RoboticFish_Maneuverability_model/State Estimates & VR Animation/Quaternions to Euler Angles ==
  Quaternions : Inport
  Add : Sum  Inputs=4
  Add{1,3..4,6} (4 alike) : Sum
  Add2 : Sum  Inputs=+-
  Add5 : Sum  Inputs=+-
  Add7 : Sum  Inputs=+-
  Constant : Constant  Value=[0; 0; 0; 0]
  Constant1 : Constant
  Constant2 : Constant
  Demux : Demux
  Demux1 : Demux
  Gain{,1..4} (5 alike) : Gain  Gain=2
  Math Function{,2..4} (4 alike) : Math  Operator=square  SignedPower=on
  Math Function1 : Math  Operator=reciprocal  SignedPower=on
  Mux : Mux  Inputs=3
  Product{,1..6} (7 alike) : Product
  Sqrt : Sqrt
  Switch : Switch  Criteria=u2 > Threshold  SaturateOnIntegerOverflow=off  InputSameDT=off
  Trigonometric Function : Trigonometry  Operator=atan2
  Trigonometric Function1 : Trigonometry  Operator=asin
  Trigonometric Function2 : Trigonometry  Operator=atan2
  Euler Angles : Outport  VectorParamsAs1DForOutWhenUnconnected=off
  wires:
  Quaternions/1 -> Product/1, Math Function/1
  Add/1 -> Sqrt/1
  Sqrt/1 -> Math Function1/1, Switch/2
  Constant/1 -> Switch/3
  Math Function1/1 -> Product/2
  Product/1 -> Switch/1
  Switch/1 -> Demux1/1
  Demux1/1 -> Product5/1, Product3/1, Product1/1  "q0"
  Demux1/2 -> Product6/1, Product4/1, Product1/2, Math Function2/1  "q1"
  Demux1/3 -> Product6/2, Product3/2, Product2/1, Math Function3/1  "q2"
  Demux1/4 -> Product5/2, Product4/2, Product2/2, Math Function4/1  "q3"
  Trigonometric Function1/1 -> Mux/2
  Mux/1 -> Euler Angles/1
  Trigonometric Function/1 -> Mux/1
  Trigonometric Function2/1 -> Mux/3
  Gain/1 -> Trigonometric Function/1
  Gain1/1 -> Trigonometric Function2/1
  Gain2/1 -> Trigonometric Function1/1
  Add1/1 -> Gain/1
  Add2/1 -> Gain2/1
  Add3/1 -> Gain1/1
  Product3/1 -> Add2/1
  Product4/1 -> Add2/2
  Product5/1 -> Add3/1
  Product6/1 -> Add3/2
  Product2/1 -> Add1/2
  Product1/1 -> Add1/1
  Add4/1 -> Gain3/1
  Gain3/1 -> Add5/2
  Constant1/1 -> Add5/1
  Add5/1 -> Trigonometric Function/2
  Add7/1 -> Trigonometric Function2/2
  Add6/1 -> Gain4/1
  Gain4/1 -> Add7/2
  Constant2/1 -> Add7/1
  Math Function2/1 -> Add4/1
  Math Function3/1 -> Add6/1, Add4/2
  Math Function4/1 -> Add6/2
  Demux/1 -> Add/1
  Demux/2 -> Add/2
  Demux/3 -> Add/3
  Demux/4 -> Add/4
  Math Function/1 -> Demux/1

== system RoboticFish_Maneuverability_model/State Estimates & VR Animation/VR sink ==
  uCMD : Inport
  eta_N : Inport  Port=2
  Bus Selector : BusSelector  OutputSignals=uHT2,uHT1,uVT1,uHT3_1,uHT3_2,uHT3_3,uVT2,uVT3
  RF Position and Rotation to VR Translation and Rotation : Subsystem
  T_ rotation : Subsystem
  To Multimedia File : dspvision/To Multimedia File  outputFilename=output.mp4  streamSelection=Video only  videoCompressor=None (uncompressed)  audioCompressor=None (uncompressed)  imagePorts=One multidimensional signal  fileType=MPEG4  audioDatatype=Determine from input data type  fourcc=RGB  videoQuality=100  mj2000CompFactor=10
      settings: LibrarySourceBlock=visionsinks/To Multimedia File
  VR To Video : vrlib/VR To Video  InstantiateOnLoad=on  SampleTime=0.1  ViewEnable=on  RemoteChange=off  RemoteView=off  FieldsWritten=RF_Gem.rotation.4.1.1.double#RF_Gem.translation.3.1.1.double#RightPaddle.rotation.4.1.1.double#LeftPaddle.rotation.4.1.1.double#CenterPaddle.rotation.4.1.1.double#Joint1.rotation.4.1.1.double#Joint2.rotation.4.1.1.double#Joint3.rotation.4.1.1.double#LeftFin.rotation.4.1.1.double#RightFin.rotation.4.1.1.double  WorldFileName=Final_HDF.wrl  AutoView=on  VideoDimensions=[200 320]  AllowVariableSize=off  FigureProperties="{'Position', 'Name', 'Viewpoint', 'CameraBound', 'CameraDirection', 'CameraPosition', 'CameraUpVector', 'ZoomFactor', 'Antialiasing', 'Headlight', 'Lighting', 'NavPanel', 'Sound', 'StatusBar', 'Stereo3D', 'Stereo3DCameraOffset', 'Stereo3DHIT', 'ToolBar', 'Textures', 'Transparency', 'Triad', 'Wireframe', 'NavZones', 'NavMode', 'NavSpeed', 'CaptureFileFormat', 'CaptureFileName', 'Record2DCompressMethod', 'Record2DCompressQuality', 'Record2D', 'Record2DFileName', 'Record2DFPS'; [5.0000000000000000e+00   9.2000000000000000e+01   5.7600000000000000e+02   3.5000000000000000e+02], '', 'Camera1-SOUTH', 'on', [0.0000000000000000e+00   0.0000000000000000e+00  -1.0000000000000000e+00], [0.0000000000000000e+00   0.0000000000000000e+00   0.0000000000000000e+00], [0.0000000000000000e+00   1.0000000000000000e+00   0.0000000000000000e+00], [1.0000000000000000e+00], 'on', 'on', 'on', 'halfbar', 'on', 'on', 'off', [1.0000000149011612e-01], [0.0000000000000000e+00], 'on', 'on', 'on', 'none', 'off', 'off', 'fly', 'normal', 'tif', '%f_anim_%n.tif', 'auto', [7.5000000000000000e+01], 'off', '%f_anim_%n.avi', 'auto'}"
  wires:
  T_ rotation/1(T_rotation) -> Bus Selector/1
  uCMD/1 -> T_ rotation/1(uCMD)
  eta_N/1 -> RF Position and Rotation to VR Translation and Rotation/1(eta_N)
  RF Position and Rotation to VR Translation and Rotation/1(VR Rotation) -> VR To Video/1
  RF Position and Rotation to VR Translation and Rotation/2(VR Translation) -> VR To Video/2
  Bus Selector/1 -> VR To Video/3  "<uHT2>"
  Bus Selector/2 -> VR To Video/4  "<uHT1>"
  Bus Selector/3 -> VR To Video/5  "<uVT1>"
  Bus Selector/4 -> VR To Video/6  "<uHT3_1>"
  Bus Selector/5 -> VR To Video/7  "<uHT3_2>"
  Bus Selector/6 -> VR To Video/8  "<uHT3_3>"
  Bus Selector/7 -> VR To Video/9  "<uVT2>"
  Bus Selector/8 -> VR To Video/10  "<uVT3>"
  VR To Video/1 -> To Multimedia File/1

== system RoboticFish_Maneuverability_model/State Estimates & VR Animation/signal transformation1 ==
  Position : Inport
  nu_B : Inport  Port=2
  Bus Creator : BusCreator  Inputs=6
  Bus Creator1 : BusCreator  Inputs=6
  Bus Creator2 : BusCreator  Inputs=2
  Selector : Selector  InputPortWidth=6  IndexOptions=Index vector (dialog)  Indices=[1]  OutputSizes=1
  Selector1 : Selector  InputPortWidth=6  IndexOptions=Index vector (dialog)  Indices=[2]  OutputSizes=1
  Selector10 : Selector  InputPortWidth=6  IndexOptions=Index vector (dialog)  Indices=[5]  OutputSizes=1
  Selector11 : Selector  InputPortWidth=6  IndexOptions=Index vector (dialog)  Indices=[6]  OutputSizes=1
  Selector2 : Selector  InputPortWidth=6  IndexOptions=Index vector (dialog)  Indices=[3]  OutputSizes=1
  Selector3 : Selector  InputPortWidth=6  IndexOptions=Index vector (dialog)  Indices=[4]  OutputSizes=1
  Selector4 : Selector  InputPortWidth=6  IndexOptions=Index vector (dialog)  Indices=[5]  OutputSizes=1
  Selector5 : Selector  InputPortWidth=6  IndexOptions=Index vector (dialog)  Indices=[6]  OutputSizes=1
  Selector6 : Selector  InputPortWidth=6  IndexOptions=Index vector (dialog)  Indices=[1]  OutputSizes=1
  Selector7 : Selector  InputPortWidth=6  IndexOptions=Index vector (dialog)  Indices=[2]  OutputSizes=1
  Selector8 : Selector  InputPortWidth=6  IndexOptions=Index vector (dialog)  Indices=[3]  OutputSizes=1
  Selector9 : Selector  InputPortWidth=6  IndexOptions=Index vector (dialog)  Indices=[4]  OutputSizes=1
  State Estimate : Outport  VectorParamsAs1DForOutWhenUnconnected=off
  wires:
  Position/1 -> Selector5/1, Selector4/1, Selector3/1, Selector2/1, Selector1/1, Selector/1
  Selector/1 -> Bus Creator/1  "X"
  Selector1/1 -> Bus Creator/2  "Y"
  Selector2/1 -> Bus Creator/3  "Z"
  Selector3/1 -> Bus Creator/4  "Roll"
  Selector4/1 -> Bus Creator/5  "Pitch"
  nu_B/1 -> Selector8/1, Selector7/1, Selector6/1, Selector11/1, Selector10/1, Selector9/1
  Selector6/1 -> Bus Creator1/1  "u"
  Selector7/1 -> Bus Creator1/2  "v"
  Selector8/1 -> Bus Creator1/3  "w"
  Selector9/1 -> Bus Creator1/4  "p"
  Selector10/1 -> Bus Creator1/5  "q"
  Selector11/1 -> Bus Creator1/6  "r"
  Bus Creator/1 -> Bus Creator2/1  "Position"
  Bus Creator1/1 -> Bus Creator2/2  "Velocity"
  Bus Creator2/1 -> State Estimate/1
  Selector5/1 -> Bus Creator/6  "Yaw"

== system RoboticFish_Maneuverability_model/ALL SCOPE/Subsystem/J1 ==
  eta2 : Inport
  Matrix Multiply : Product  Inputs=3  Multiplication=Matrix(*)
  Selector1 : Selector  InputPortWidth=3  IndexOptions=Index vector (dialog)  Indices=[2]  OutputSizes=1
  Selector2 : Selector  InputPortWidth=3  IndexOptions=Index vector (dialog)  Indices=[3]  OutputSizes=1
  Selector3 : Selector  InputPortWidth=3  IndexOptions=Index vector (dialog)  Indices=[1]  OutputSizes=1
  Subsystem : Subsystem
  Subsystem1 : Subsystem
  Subsystem2 : Subsystem
  J1 : Outport
  wires:
  Selector1/1 -> Subsystem1/1(Pitch)  "Pitch"
  eta2/1 -> Selector3/1, Selector2/1, Selector1/1
  Selector2/1 -> Subsystem2/1(Yaw)  "Yaw"
  Selector3/1 -> Subsystem/1(Roll)  "Roll"
  Subsystem1/1(Cy,Pitch) -> Matrix Multiply/2
  Subsystem/1(Cx,Roll) -> Matrix Multiply/1
  Subsystem2/1(Cz,Yaw) -> Matrix Multiply/3
  Matrix Multiply/1 -> J1/1

== system RoboticFish_Maneuverability_model/ALL SCOPE/Subsystem/J2 ==
  eta2 : Inport
  Constant : Constant
  Constant1 : Constant  Value=0
  Create 3x3 Matrix : sharedutil/Create 3x3 Matrix  aMode=aMode
  Divide : Product  Inputs=*/
  Divide1 : Product  Inputs=*/
  Gain : Gain  Gain=-1
  Product : Product
  Product1 : Product
  Selector1 : Selector  InputPortWidth=3  IndexOptions=Index vector (dialog)  Indices=[2]  OutputSizes=1
  Selector3 : Selector  InputPortWidth=3  IndexOptions=Index vector (dialog)  Indices=[1]  OutputSizes=1
  SinCos : Trigonometry  Operator=sincos
  SinCos1 : Trigonometry  Operator=tan
  SinCos2 : Trigonometry  Operator=cos
  J2 : Outport
  wires:
  Selector3/1 -> SinCos/1  "Roll"
  eta2/1 -> Selector1/1, Selector3/1
  Selector1/1 -> SinCos1/1, SinCos2/1  "Pitch"
  SinCos/1 -> Divide/1, Gain/1, Product/1  "sin(Roll)"
  SinCos2/1 -> Divide1/2, Divide/2  "cos(Pitch)"
  SinCos1/1 -> Product1/2, Product/2  "tan(Pitch)"
  SinCos/2 -> Create 3x3 Matrix/5, Divide1/1, Product1/1  "cos(Roll)"
  Product/1 -> Create 3x3 Matrix/2  "sin(Roll)*tan(Pitch)"
  Product1/1 -> Create 3x3 Matrix/3  "cos(Roll)*tan(Pitch)"
  Divide/1 -> Create 3x3 Matrix/8  "sin(Roll)/cos(Pitch)"
  Divide1/1 -> Create 3x3 Matrix/9  "cos(Roll)/cos(Pitch)"
  Constant/1 -> Create 3x3 Matrix/1
  Constant1/1 -> Create 3x3 Matrix/7, Create 3x3 Matrix/4
  Gain/1 -> Create 3x3 Matrix/6
  Create 3x3 Matrix/1 -> J2/1

== system RoboticFish_Maneuverability_model/Control parameter input/Subsystem/Saturation limits ==
  InBus : Inport
  Bus Creator : BusCreator  Inputs=7
  Saturation Thetastr_HT3 : Saturate  UpperLimit=pi/4  LowerLimit=-pi/4
  Saturation f_HT3 : Saturate  UpperLimit=2  LowerLimit=0
  Saturation uHT1 : Saturate  UpperLimit=30  LowerLimit=-30
  Saturation uHT2 : Saturate  UpperLimit=30  LowerLimit=-30
  Saturation uVT1 : Saturate  UpperLimit=15  LowerLimit=-15
  Saturation uVT2 : Saturate  UpperLimit=pi/3  LowerLimit=-pi/3
  Saturation uVT3 : Saturate  UpperLimit=pi/3  LowerLimit=-pi/3
  Selector Thetastr_HT3 : Selector  InputPortWidth=7  IndexOptions=Index vector (dialog)  Indices=[5]  OutputSizes=1
  Selector f_HT3 : Selector  InputPortWidth=7  IndexOptions=Index vector (dialog)  Indices=[4]  OutputSizes=1
  Selector uHT1 : Selector  InputPortWidth=7  IndexOptions=Index vector (dialog)  Indices=[1]  OutputSizes=1
  Selector uHT2 : Selector  InputPortWidth=7  IndexOptions=Index vector (dialog)  Indices=[2]  OutputSizes=1
  Selector uVT1 : Selector  InputPortWidth=7  IndexOptions=Index vector (dialog)  Indices=[3]  OutputSizes=1
  Selector uVT3 : Selector  InputPortWidth=7  IndexOptions=Index vector (dialog)  Indices=[7]  OutputSizes=1
  Selector5 uVT2 : Selector  InputPortWidth=7  IndexOptions=Index vector (dialog)  Indices=[6]  OutputSizes=1
  uCMD : Outport  VectorParamsAs1DForOutWhenUnconnected=off
  wires:
  Saturation uVT3/1 -> Bus Creator/7  "uVT3"
  Saturation uVT2/1 -> Bus Creator/6  "uVT2"
  Saturation uVT1/1 -> Bus Creator/5  "uVT1"
  Saturation uHT2/1 -> Bus Creator/4  "uHT2"
  Selector uHT1/1 -> Saturation uHT1/1
  Saturation uHT1/1 -> Bus Creator/3  "uHT1"
  Selector Thetastr_HT3/1 -> Saturation Thetastr_HT3/1
  Saturation f_HT3/1 -> Bus Creator/1  "f_HT3"
  Bus Creator/1 -> uCMD/1
  Selector uVT3/1 -> Saturation uVT3/1
  Selector5 uVT2/1 -> Saturation uVT2/1
  Selector uVT1/1 -> Saturation uVT1/1
  Selector uHT2/1 -> Saturation uHT2/1
  InBus/1 -> Selector f_HT3/1, Selector Thetastr_HT3/1, Selector uHT1/1, Selector uHT2/1, Selector5 uVT2/1, Selector uVT3/1, Selector uVT1/1
  Saturation Thetastr_HT3/1 -> Bus Creator/2  "Thetastr_HT3"
  Selector f_HT3/1 -> Saturation f_HT3/1

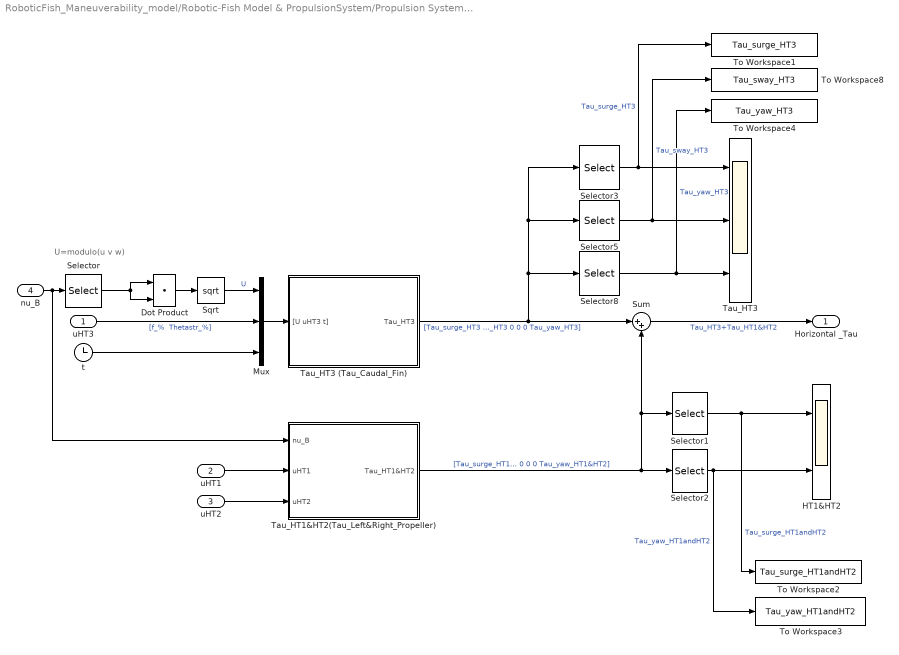
== system RoboticFish_Maneuverability_model/Robotic-Fish Model & PropulsionSystem/Propulsion System/Horizontal Force and Moment (Tau_H) ==
  note: U=modulo(u v w)
  uHT3 : Inport
  uHT1 : Inport  Port=2
  uHT2 : Inport  Port=3
  nu_B : Inport  Port=4
  Dot Product : DotProduct  OutDataTypeStr=Inherit: Inherit via internal rule
  HT1&HT2 : Scope  NumInputPorts=2
  Mux : Mux  Inputs=3
  Selector : Selector  InputPortWidth=6  IndexOptions=Index vector (dialog)  Indices=[1 2 3]  OutputSizes=1
  Selector1 : Selector  InputPortWidth=6  IndexOptions=Index vector (dialog)  Indices=[1]  OutputSizes=1
  Selector2 : Selector  InputPortWidth=6  IndexOptions=Index vector (dialog)  Indices=[6]  OutputSizes=1
  Selector3 : Selector  InputPortWidth=6  IndexOptions=Index vector (dialog)  Indices=[1]  OutputSizes=1
  Selector5 : Selector  InputPortWidth=6  IndexOptions=Index vector (dialog)  Indices=[2]  OutputSizes=1
  Selector8 : Selector  InputPortWidth=6  IndexOptions=Index vector (dialog)  Indices=[6]  OutputSizes=1
  Sqrt : Sqrt
  Sum : Sum  Inputs=|++
  Tau_HT1&HT2(Tau_Left&Right_Propeller) : Subsystem
  Tau_HT3 : Scope  NumInputPorts=3
  Tau_HT3 (Tau_Caudal_Fin) : Subsystem
  To Workspace1 : ToWorkspace  VariableName=Tau_surge_HT3  SampleTime=-1
  To Workspace2 : ToWorkspace  VariableName=Tau_surge_HT1andHT2  SampleTime=-1
  To Workspace3 : ToWorkspace  VariableName=Tau_yaw_HT1andHT2  SampleTime=-1
  To Workspace4 : ToWorkspace  VariableName=Tau_yaw_HT3  SampleTime=-1
  To Workspace8 : ToWorkspace  VariableName=Tau_sway_HT3  SampleTime=-1
  t : Clock
  Horizontal _Tau : Outport  VectorParamsAs1DForOutWhenUnconnected=off
  wires:
  Tau_HT3 (Tau_Caudal_Fin)/1(Tau_HT3) -> Sum/1, Selector3/1, Selector5/1, Selector8/1  "[Tau_surge_HT3 Tau_sway_HT3 0 0 0 Tau_yaw_HT3]"
  Sum/1 -> Horizontal _Tau/1  "Tau_HT3+Tau_HT1&HT2"
  nu_B/1 -> Tau_HT1&HT2(Tau_Left&Right_Propeller)/1(nu_B), Selector/1
  Selector/1 -> Dot Product/2, Dot Product/1
  Mux/1 -> Tau_HT3 (Tau_Caudal_Fin)/1("[U uHT3 t]")
  t/1 -> Mux/3
  Dot Product/1 -> Sqrt/1
  uHT3/1 -> Mux/2  "[f_%  Thetastr_%]"
  Sqrt/1 -> Mux/1  "U"
  uHT1/1 -> Tau_HT1&HT2(Tau_Left&Right_Propeller)/2(uHT1)
  uHT2/1 -> Tau_HT1&HT2(Tau_Left&Right_Propeller)/3(uHT2)
  Tau_HT1&HT2(Tau_Left&Right_Propeller)/1(Tau_HT1&HT2) -> Selector2/1, Selector1/1, Sum/2  "[Tau_surge_HT1&HT2 0 0 0 0 Tau_yaw_HT1&HT2]"
  Selector2/1 -> To Workspace3/1, HT1&HT2/2  "Tau_yaw_HT1andHT2"
  Selector5/1 -> To Workspace8/1, Tau_HT3/2  "Tau_sway_HT3"
  Selector3/1 -> To Workspace1/1, Tau_HT3/1  "Tau_surge_HT3"
  Selector8/1 -> To Workspace4/1, Tau_HT3/3  "Tau_yaw_HT3"
  Selector1/1 -> To Workspace2/1, HT1&HT2/1  "Tau_surge_HT1andHT2"

== system RoboticFish_Maneuverability_model/Robotic-Fish Model & PropulsionSystem/Propulsion System/Vertical Force and Moment (Tau_V) ==
  note: Tau_VT2&VT3= [ 0 Ys Zs Ks Ms Ns ]
  note: Tau_VT1=[0 0 Fvt1 0 Tvt1 0 ]
  nu_B : Inport
  uVT1 : Inport  Port=2
  "[uVT2 uVT3]" : Inport  Port=3
  Bus Selector : BusSelector  OutputSignals=uVT2,uVT3
  Selector : Selector  InputPortWidth=6  IndexOptions=Index vector (dialog)  Indices=[1]  OutputSizes=1
  Selector1 : Selector  InputPortWidth=6  IndexOptions=Index vector (dialog)  Indices=[4]  OutputSizes=1
  Selector10 : Selector  InputPortWidth=6  IndexOptions=Index vector (dialog)  Indices=[5]  OutputSizes=1
  Selector2 : Selector  InputPortWidth=6  IndexOptions=Index vector (dialog)  Indices=[2]  OutputSizes=1
  Selector3 : Selector  InputPortWidth=6  IndexOptions=Index vector (dialog)  Indices=[3]  OutputSizes=1
  Selector4 : Selector  InputPortWidth=6  IndexOptions=Index vector (dialog)  Indices=[5]  OutputSizes=1
  Selector5 : Selector  InputPortWidth=6  IndexOptions=Index vector (dialog)  Indices=[6]  OutputSizes=1
  Selector9 : Selector  InputPortWidth=6  IndexOptions=Index vector (dialog)  Indices=[3]  OutputSizes=1
  Sum : Sum  Inputs=|++
  Tau_VT1 : Scope  NumInputPorts=2
  Tau_VT1 (Tau_Middle_Propeller) : Subsystem
  Tau_VT2&VT3 : Scope  NumInputPorts=6
  Tau_VT2&VT3 (Tau_Pectoral Fin) : Subsystem
  To Workspace1 : ToWorkspace  VariableName=Tau_heave_VT2andVT3  SampleTime=-1
  To Workspace2 : ToWorkspace  VariableName=Tau_pitch_VT1  SampleTime=-1
  To Workspace3 : ToWorkspace  VariableName=Tau_pitch_VT2andVT3  SampleTime=-1
  To Workspace4 : ToWorkspace  VariableName=Tau_heave_VT1  SampleTime=-1
  To Workspace5 : ToWorkspace  VariableName=Tau_roll_VT2andVT3  SampleTime=-1
  Vertical_Tau : Outport  VectorParamsAs1DForOutWhenUnconnected=off
  wires:
  Sum/1 -> Vertical_Tau/1
  "[uVT2 uVT3]"/1 -> Bus Selector/1
  Bus Selector/1 -> Tau_VT2&VT3 (Tau_Pectoral Fin)/1("uVT2 ")  "<uVT2>"
  Bus Selector/2 -> Tau_VT2&VT3 (Tau_Pectoral Fin)/2(uVT3)  "<uVT3>"
  nu_B/1 -> Tau_VT1 (Tau_Middle_Propeller)/1(nu_B), Tau_VT2&VT3 (Tau_Pectoral Fin)/3(nu_B)
  uVT1/1 -> Tau_VT1 (Tau_Middle_Propeller)/2(uVT1)
  Selector4/1 -> To Workspace3/1, Tau_VT2&VT3/5  "Tau_pitch_VT2&VT3"
  Tau_VT2&VT3 (Tau_Pectoral Fin)/1("tau_VT2 & tau_VT3 ") -> Sum/1, Selector/1, Selector2/1, Selector3/1, Selector1/1, Selector4/1, Selector5/1
  Selector1/1 -> To Workspace5/1, Tau_VT2&VT3/4  "Tau_roll_VT2&VT3"
  Selector2/1 -> Tau_VT2&VT3/2  "Tau_sway_VT2&VT3"
  Selector/1 -> Tau_VT2&VT3/1  "Tau_surge_VT2&VT3"
  Selector5/1 -> Tau_VT2&VT3/6  "Tau_yaw_VT2&VT3"
  Selector3/1 -> To Workspace1/1, Tau_VT2&VT3/3  "Tau_heave_VT2&VT3"
  Tau_VT1 (Tau_Middle_Propeller)/1(Tau_VT1) -> Sum/2, Selector10/1, Selector9/1
  Selector10/1 -> To Workspace2/1, Tau_VT1/2  "Tau_pitch_VT1"
  Selector9/1 -> To Workspace4/1, Tau_VT1/1  "Tau_heave_VT1"
